simulink model "lab4z"  (Simulink 4.00)
settings: Solver=ode45  StartTime=0.0  StopTime=10.0  RelTol=1e-3
libraries: cstblocks x2
settings Model: LastModifiedBy=daemok

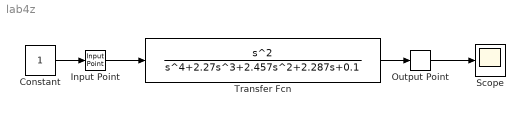
== system lab4z ==
  Constant : Constant  Value=1
  Input Point : cstblocks/Input Point
  Output Point : cstblocks/Output Point
  Scope : Scope
      settings: TimeRange=auto  YMin=-5  YMax=5  SaveToWorkspace=off  SaveName=ScopeData  LimitDataPoints=on  MaxDataPoints=5000
  Transfer Fcn : TransferFcn  Numerator=[1 0 0]  Denominator=[1 2.27 2.457 2.287 0.1]  AbsoluteTolerance=auto  Realization=auto
  wires:
  Constant/1 -> Input Point/1
  Input Point/1 -> Transfer Fcn/1
  Transfer Fcn/1 -> Output Point/1
  Output Point/1 -> Scope/1
